simulink model "manipulacion_1_enlace"  (R2022b)
settings: Solver=VariableStepAuto  StartTime=0.0  StopTime=30  RelTol=1e-3
settings Model: Creator=alex  LastModifiedBy=alex

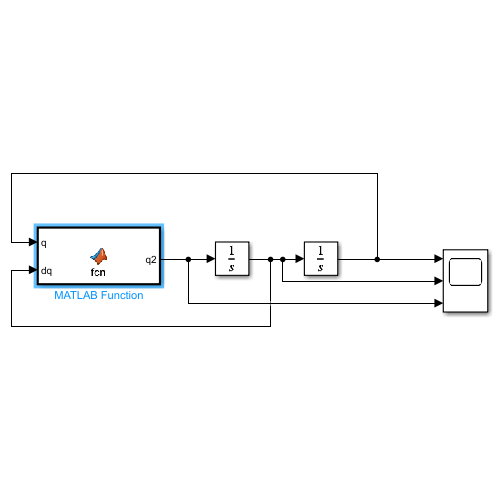
[thumbnail: Simulink's stored preview of the top-level diagram]
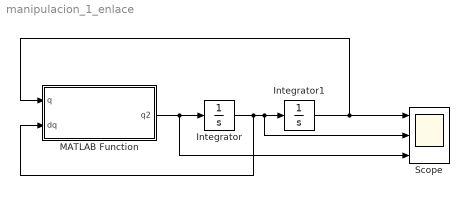
== system manipulacion_1_enlace ==
  Integrator : Integrator
  Integrator1 : Integrator
  MATLAB Function : MATLAB Function  TreatAsAtomicUnit=on
  Scope : Scope  NumInputPorts=3
  wires:
  Integrator1/1 -> MATLAB Function/1(q), Scope/1
  Integrator/1 -> MATLAB Function/2(dq), Scope/2, Integrator1/1
  MATLAB Function/1(q2) -> Scope/3, Integrator/1

== matlab function manipulacion_1_enlace/MATLAB Function ==
  data: q input; q2 output; dq input
function q2 = fcn(q,dq)


k=0.01;
m = 5;
l=0.36
g=9.8
t = 0.0
a= l/2
j=(4/3)*(m*a*a)


q2= (-(m*g*a*cos(q))+t-(k*dq))/j
